simulink model "test"  (R2021a)
settings: Solver=FixedStepAuto  StartTime=0.0  StopTime=inf  RelTol=1e-3
libraries: robotlib x2
settings Model: Creator=ACER  LastModifiedBy=tarun
settings OptimizationCC: EnhancedBackFolding=on  PassReuseOutputArgsAs=Individual arguments  ZeroExternalMemoryAtStartup=off  ZeroInternalMemoryAtStartup=off  MaxStackSize=64  OptimizeBlockOrder=speed  DifferentSizesBufferReuse=on  OptimizationCustomize=off  EfficientTunableParamExpr=on
settings DebuggingCC: ParameterTunabilityLossMsg=error
settings HardwareCC: ProdBitPerPointer=32  ProdBitPerSizeT=32  ProdBitPerPtrDiffT=32  ProdLargestAtomicFloat=None  ProdIntDivRoundTo=Undefined  ProdEndianess=Unspecified  ProdWordSize=32  ProdHWDeviceType=Generic->Unspecified (assume 32-bit Generic)
settings SFSimCC: MATLABDynamicMemAlloc=off
settings RTWCC: SystemTargetFile=ert.tlc  HardwareBoard=Robot Operating System (ROS)  TLCOptions="-aInlineSetEventsForThisBaseRateFcn=TLC_FALSE -aSuppressMultiTaskScheduler=TLC_FALSE  -aRateBasedStepFcn=0"  TemplateMakefile=ert_default_tmf  Toolchain=Catkin  TargetLang=C++
settings CodeAppCC: ForceParamTrailComments=on  IgnoreCustomStorageClasses=off  OperatorAnnotations=on  SimulinkDataObjDesc=on  SFDataObjDesc=on  InsertBlockDesc=on

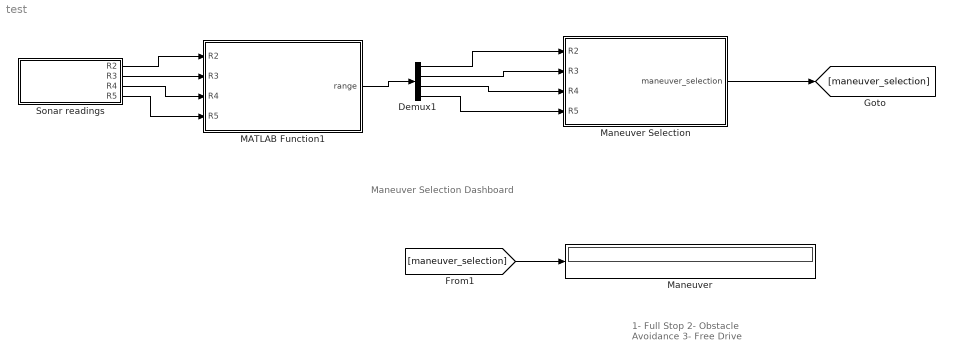
== system test ==
  note: 1- Full Stop
      | 2- Obstacle Avoidance
      | 3- Free Drive
  note: Maneuver Selection Dashboard
  Demux1 : Demux
  MATLAB Function1 : MATLAB Function  TreatAsAtomicUnit=on
  Maneuver : Display
  Maneuver Selection : Stateflow chart  TreatAsAtomicUnit=on
  Sonar readings : Subsystem
  wires:
  Demux1/4 -> Maneuver Selection/4(R5)
  MATLAB Function1/1(range) -> Demux1/1
  Demux1/3 -> Maneuver Selection/3(R4)
  [maneuver_selection] -> Maneuver/1
  Maneuver Selection/1(maneuver_selection) -> [maneuver_selection]
  Demux1/1 -> Maneuver Selection/1(R2)
  Demux1/2 -> Maneuver Selection/2(R3)
  Sonar readings/1(R2) -> MATLAB Function1/1(R2)
  Sonar readings/2(R3) -> MATLAB Function1/2(R3)
  Sonar readings/3(R4) -> MATLAB Function1/3(R4)
  Sonar readings/4(R5) -> MATLAB Function1/4(R5)

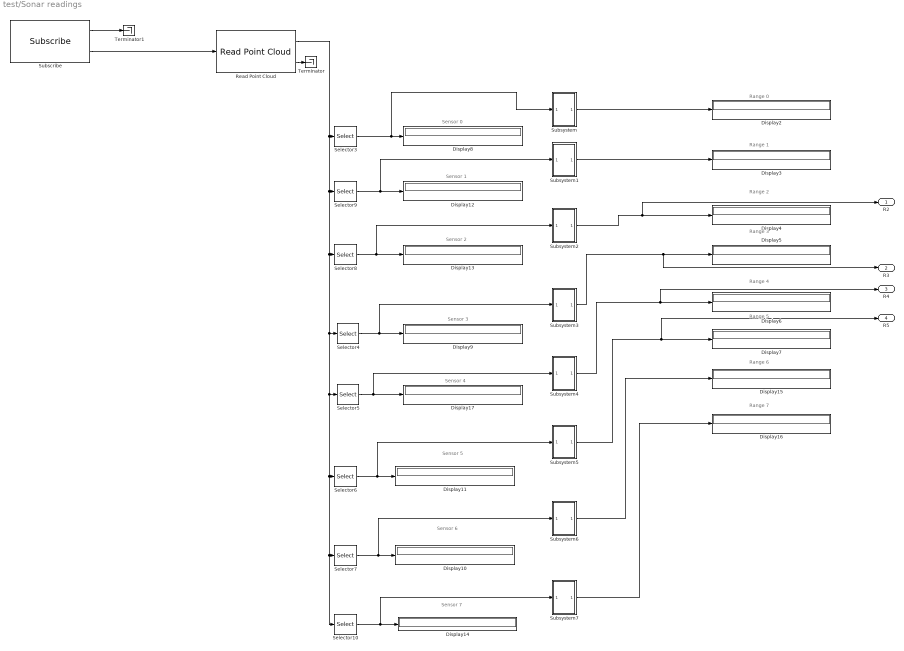
== system test/Sonar readings ==
  note: Range 3
  note: Range 5
  note: Sensor 7
  note: Sensor 6
  note: Range 0
  note: Sensor 0
  note: Range 2
  note: Range 4
  note: Range 6
  note: Range 7
  note: Sensor 2
  note: Sensor 3
  note: Sensor 5
  note: Range 1
  note: Sensor 4
  note: Sensor 1
  Display{2..17} (16 alike) : Display
  Read Point Cloud : robotlib/Read Point Cloud  MaximumPointCloudSize=[8, 1]  PreserveStructure=off  ShowRGBOutput=off  ShowIntensityOutput=off  ShowErrorCodeOutput=on  VariableSizeOutputs=off
      settings: SourceProductBaseCode=RR
  Selector10 : Selector  NumberOfDimensions=2  InputPortWidth=6  IndexOptions=Starting index (dialog),Starting index (dialog)  Indices=8,1  OutputSizes=1,3
  Selector3 : Selector  NumberOfDimensions=2  InputPortWidth=6  IndexOptions=Starting index (dialog),Starting index (dialog)  Indices=1,1  OutputSizes=1,3
  Selector4 : Selector  NumberOfDimensions=2  InputPortWidth=6  IndexOptions=Starting index (dialog),Starting index (dialog)  Indices=4,1  OutputSizes=1,3
  Selector5 : Selector  NumberOfDimensions=2  InputPortWidth=6  IndexOptions=Starting index (dialog),Starting index (dialog)  Indices=5,1  OutputSizes=1,3
  Selector6 : Selector  NumberOfDimensions=2  InputPortWidth=6  IndexOptions=Starting index (dialog),Starting index (dialog)  Indices=6,1  OutputSizes=1,3
  Selector7 : Selector  NumberOfDimensions=2  InputPortWidth=6  IndexOptions=Starting index (dialog),Starting index (dialog)  Indices=7,1  OutputSizes=1,3
  Selector8 : Selector  NumberOfDimensions=2  InputPortWidth=6  IndexOptions=Starting index (dialog),Starting index (dialog)  Indices=3,1  OutputSizes=1,3
  Selector9 : Selector  NumberOfDimensions=2  InputPortWidth=6  IndexOptions=Starting index (dialog),Starting index (dialog)  Indices=2,1  OutputSizes=1,3
  Subscribe : robotlib/Subscribe  topicSource=Select from ROS network  topic=/RosAria/sonar_pointcloud2  messageType=sensor_msgs/PointCloud2  SampleTime=0.05  legacyBusStruct=off  messageQueueLength=1
  Subsystem : Subsystem
  Subsystem1 : Subsystem
  Subsystem2 : Subsystem
  Subsystem3 : Subsystem
  Subsystem4 : Subsystem
  Subsystem5 : Subsystem
  Subsystem6 : Subsystem
  Subsystem7 : Subsystem
  Terminator : Terminator
  Terminator1 : Terminator
  R2 : Outport
  R3 : Outport  Port=2
  R4 : Outport  Port=3
  R5 : Outport  Port=4
  wires:
  Subscribe/2 -> Read Point Cloud/1
  Subscribe/1 -> Terminator1/1
  Selector7/1 -> Subsystem6/1(In1), Display10/1
  Read Point Cloud/1 -> Selector3/1, Selector9/1, Selector8/1, Selector4/1, Selector5/1, Selector6/1, Selector10/1, Selector7/1
  Subsystem5/1(Out1) -> R5/1, Display7/1
  Subsystem4/1(Out1) -> R4/1, Display6/1
  Subsystem3/1(Out1) -> R3/1, Display5/1
  Selector8/1 -> Subsystem2/1(In1), Display13/1
  Selector4/1 -> Subsystem3/1(In1), Display9/1
  Subsystem/1(Out1) -> Display2/1
  Selector9/1 -> Subsystem1/1(In1), Display12/1
  Selector5/1 -> Subsystem4/1(In1), Display17/1
  Read Point Cloud/2 -> Terminator/1
  Selector10/1 -> Subsystem7/1(In1), Display14/1
  Selector6/1 -> Subsystem5/1(In1), Display11/1
  Subsystem1/1(Out1) -> Display3/1
  Subsystem7/1(Out1) -> Display16/1
  Subsystem6/1(Out1) -> Display15/1
  Selector3/1 -> Display8/1, Subsystem/1(In1)
  Subsystem2/1(Out1) -> R2/1, Display4/1

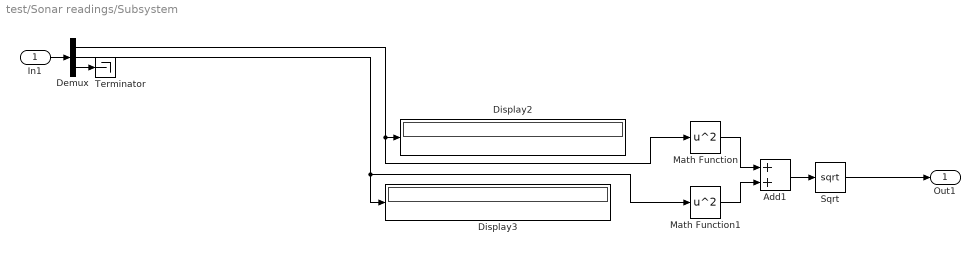
== system test/Sonar readings/Subsystem ==
  In1 : Inport
  Add1 : Sum
  Demux : Demux  Outputs=3
  Display2 : Display
  Display3 : Display
  Math Function : Math  Operator=square  SaturateOnIntegerOverflow=on
  Math Function1 : Math  Operator=square  SaturateOnIntegerOverflow=on
  Sqrt : Sqrt  SaturateOnIntegerOverflow=on
  Terminator : Terminator
  Out1 : Outport
  wires:
  Math Function1/1 -> Add1/2
  Demux/1 -> Math Function/1, Display2/1
  In1/1 -> Demux/1
  Math Function/1 -> Add1/1
  Demux/2 -> Display3/1, Math Function1/1
  Sqrt/1 -> Out1/1
  Add1/1 -> Sqrt/1
  Demux/3 -> Terminator/1

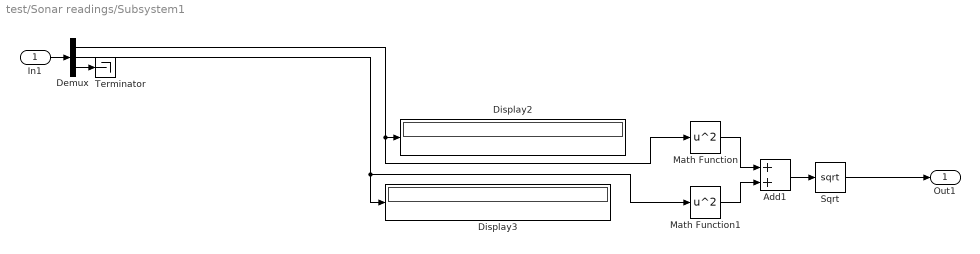
== system test/Sonar readings/Subsystem1 ==
  In1 : Inport
  Add1 : Sum
  Demux : Demux  Outputs=3
  Display2 : Display
  Display3 : Display
  Math Function : Math  Operator=square  SaturateOnIntegerOverflow=on
  Math Function1 : Math  Operator=square  SaturateOnIntegerOverflow=on
  Sqrt : Sqrt  SaturateOnIntegerOverflow=on
  Terminator : Terminator
  Out1 : Outport
  wires:
  Math Function1/1 -> Add1/2
  Demux/1 -> Math Function/1, Display2/1
  In1/1 -> Demux/1
  Math Function/1 -> Add1/1
  Demux/2 -> Display3/1, Math Function1/1
  Sqrt/1 -> Out1/1
  Add1/1 -> Sqrt/1
  Demux/3 -> Terminator/1

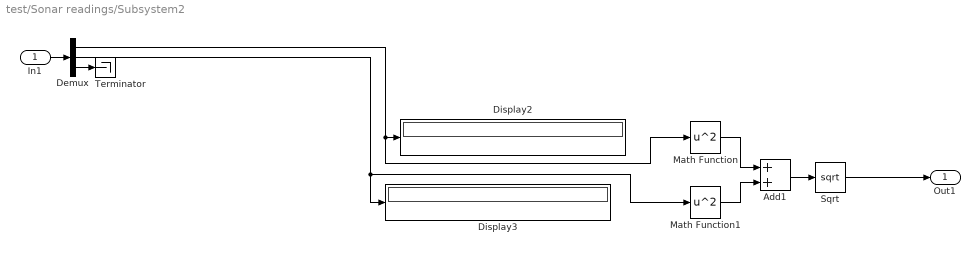
== system test/Sonar readings/Subsystem2 ==
  In1 : Inport
  Add1 : Sum
  Demux : Demux  Outputs=3
  Display2 : Display
  Display3 : Display
  Math Function : Math  Operator=square  SaturateOnIntegerOverflow=on
  Math Function1 : Math  Operator=square  SaturateOnIntegerOverflow=on
  Sqrt : Sqrt  SaturateOnIntegerOverflow=on
  Terminator : Terminator
  Out1 : Outport
  wires:
  Math Function1/1 -> Add1/2
  Demux/1 -> Math Function/1, Display2/1
  In1/1 -> Demux/1
  Math Function/1 -> Add1/1
  Demux/2 -> Display3/1, Math Function1/1
  Sqrt/1 -> Out1/1
  Add1/1 -> Sqrt/1
  Demux/3 -> Terminator/1

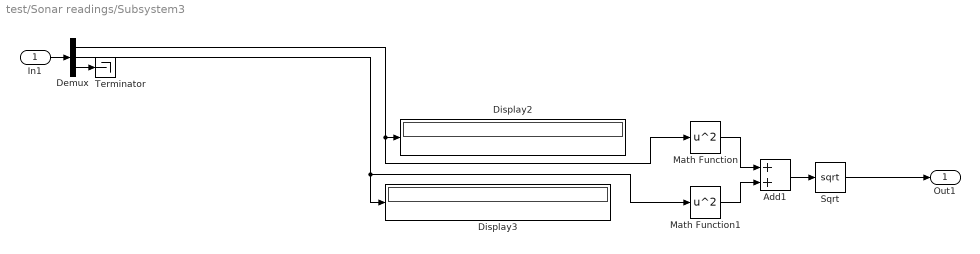
== system test/Sonar readings/Subsystem3 ==
  In1 : Inport
  Add1 : Sum
  Demux : Demux  Outputs=3
  Display2 : Display
  Display3 : Display
  Math Function : Math  Operator=square  SaturateOnIntegerOverflow=on
  Math Function1 : Math  Operator=square  SaturateOnIntegerOverflow=on
  Sqrt : Sqrt  SaturateOnIntegerOverflow=on
  Terminator : Terminator
  Out1 : Outport
  wires:
  Math Function1/1 -> Add1/2
  Demux/1 -> Math Function/1, Display2/1
  In1/1 -> Demux/1
  Math Function/1 -> Add1/1
  Demux/2 -> Display3/1, Math Function1/1
  Sqrt/1 -> Out1/1
  Add1/1 -> Sqrt/1
  Demux/3 -> Terminator/1

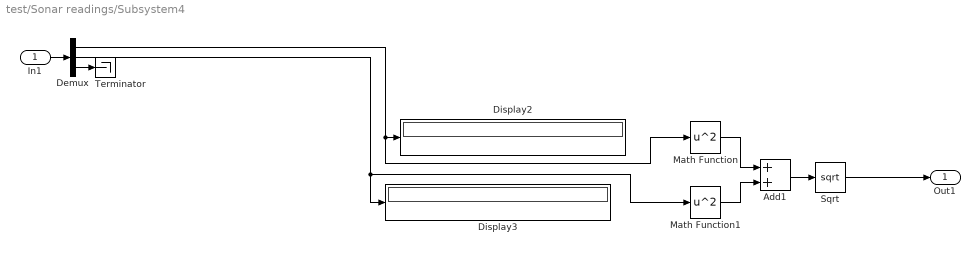
== system test/Sonar readings/Subsystem4 ==
  In1 : Inport
  Add1 : Sum
  Demux : Demux  Outputs=3
  Display2 : Display
  Display3 : Display
  Math Function : Math  Operator=square  SaturateOnIntegerOverflow=on
  Math Function1 : Math  Operator=square  SaturateOnIntegerOverflow=on
  Sqrt : Sqrt  SaturateOnIntegerOverflow=on
  Terminator : Terminator
  Out1 : Outport
  wires:
  Math Function1/1 -> Add1/2
  Demux/1 -> Math Function/1, Display2/1
  In1/1 -> Demux/1
  Math Function/1 -> Add1/1
  Demux/2 -> Display3/1, Math Function1/1
  Sqrt/1 -> Out1/1
  Add1/1 -> Sqrt/1
  Demux/3 -> Terminator/1

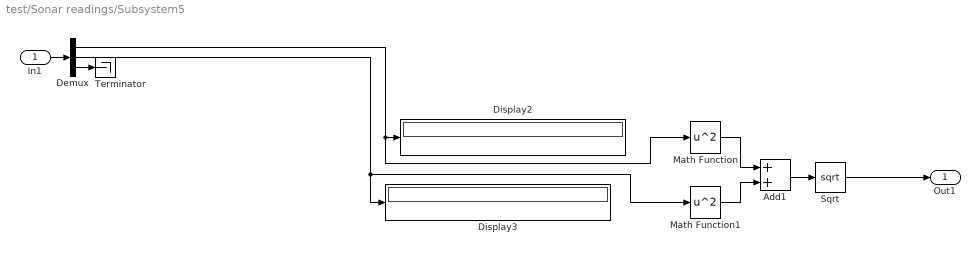
== system test/Sonar readings/Subsystem5 ==
  In1 : Inport
  Add1 : Sum
  Demux : Demux  Outputs=3
  Display2 : Display
  Display3 : Display
  Math Function : Math  Operator=square  SaturateOnIntegerOverflow=on
  Math Function1 : Math  Operator=square  SaturateOnIntegerOverflow=on
  Sqrt : Sqrt  SaturateOnIntegerOverflow=on
  Terminator : Terminator
  Out1 : Outport
  wires:
  Math Function1/1 -> Add1/2
  Demux/1 -> Math Function/1, Display2/1
  In1/1 -> Demux/1
  Math Function/1 -> Add1/1
  Demux/2 -> Display3/1, Math Function1/1
  Sqrt/1 -> Out1/1
  Add1/1 -> Sqrt/1
  Demux/3 -> Terminator/1

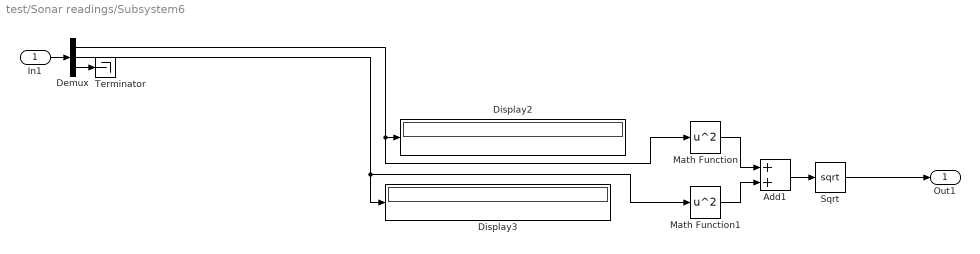
== system test/Sonar readings/Subsystem6 ==
  In1 : Inport
  Add1 : Sum
  Demux : Demux  Outputs=3
  Display2 : Display
  Display3 : Display
  Math Function : Math  Operator=square  SaturateOnIntegerOverflow=on
  Math Function1 : Math  Operator=square  SaturateOnIntegerOverflow=on
  Sqrt : Sqrt  SaturateOnIntegerOverflow=on
  Terminator : Terminator
  Out1 : Outport
  wires:
  Math Function1/1 -> Add1/2
  Demux/1 -> Math Function/1, Display2/1
  In1/1 -> Demux/1
  Math Function/1 -> Add1/1
  Demux/2 -> Display3/1, Math Function1/1
  Sqrt/1 -> Out1/1
  Add1/1 -> Sqrt/1
  Demux/3 -> Terminator/1

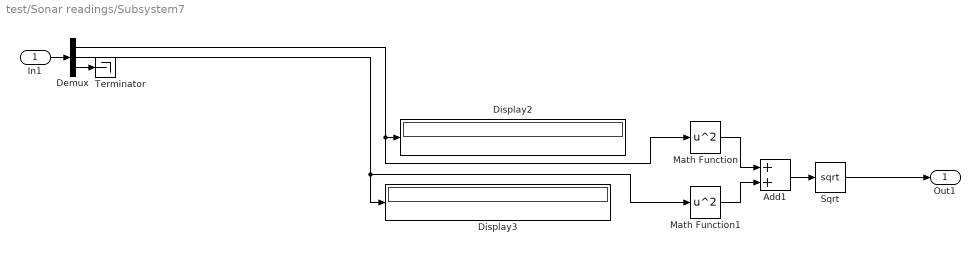
== system test/Sonar readings/Subsystem7 ==
  In1 : Inport
  Add1 : Sum
  Demux : Demux  Outputs=3
  Display2 : Display
  Display3 : Display
  Math Function : Math  Operator=square  SaturateOnIntegerOverflow=on
  Math Function1 : Math  Operator=square  SaturateOnIntegerOverflow=on
  Sqrt : Sqrt  SaturateOnIntegerOverflow=on
  Terminator : Terminator
  Out1 : Outport
  wires:
  Math Function1/1 -> Add1/2
  Demux/1 -> Math Function/1, Display2/1
  In1/1 -> Demux/1
  Math Function/1 -> Add1/1
  Demux/2 -> Display3/1, Math Function1/1
  Sqrt/1 -> Out1/1
  Add1/1 -> Sqrt/1
  Demux/3 -> Terminator/1

== stateflow chart test/Maneuver Selection ==
  (default) -> (junction 137)
  (junction 137) -> (junction 129) [order 1] : [R2 < 1 || R3 < 1 || R4 < 1 || R5 < 1]
  (junction 137) -> (junction 135) [order 2]
  (junction 129) -> (junction 138) : { maneuver_selection = 1;}
  (junction 135) -> (junction 132) [order 1] : [R2 < 2 || R3 < 2 || R4 < 2 || R5 < 2 ]
  (junction 135) -> (junction 158) [order 2] : {maneuver_selection = 3;}
  (junction 132) -> (junction 131) : {maneuver_selection = 2;}
  (junction 131) -> (junction 158)
  (junction 138) -> (junction 131)
  (junction 158) -> (junction 161)
  data: maneuver_selection output; R2 input; R3 input; R4 input; R5 input

== matlab function test/MATLAB Function1 ==
  data: range output; R2 input; R3 input; R4 input; R5 input
function range = sonarRanges(R2,R3,R4,R5)
range = [R2 R3 R4 R5];
end
